simulink model "fo_FTSM"  (R2022b)
settings: Solver=VariableStepAuto  StartTime=0.0  StopTime=10.0  RelTol=1e-3
libraries: fod x2
settings Model: Creator=张倬境  LastModifiedBy=张倬境
settings DebuggingCC: MaskedZcDiagnostic=none  IgnoredZcDiagnostic=none

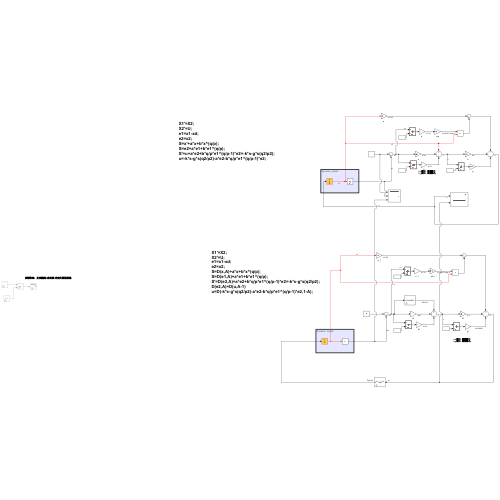
[thumbnail: Simulink's stored preview of the top-level diagram]
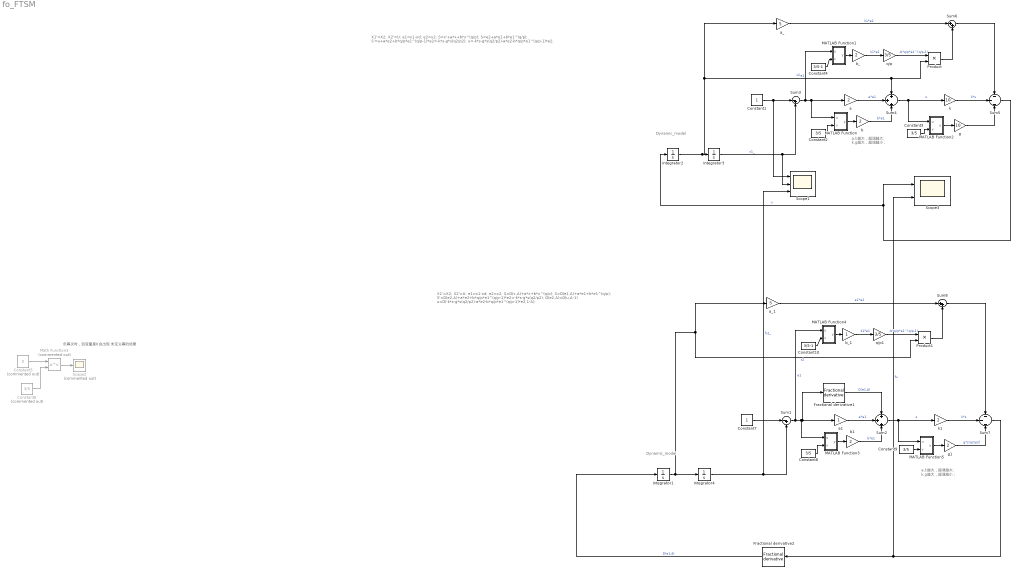
== system fo_FTSM ==
  note: a,b越大，超调越大;
      | k,g越大，超调越小；
  note: 负幂次时，自变量是0会出现 未定义幂的结果
  note: X1'=X2;
      | X2'=U;
      | e1=x1-xd;
      | e2=x2;
      | S=x'+a*x+b*x^(q/p);
      | S=e2+a*e1+b*e1^(q/p);
      | S'=u+a*e2+b*q/p*e1^(q/p-1)*e2=-k*s-g*s(q2/p2);
      | u=-k*s-g*s(q2/p2)-a*e2-b*q/p*e1^(q/p-1)*e2;
  note: Dynamic_model
  note: Dynamic_model
  note: a,b越大，超调越大;
      | k,g越大，超调越小；
  note: X1'=X2;
      | X2'=U;
      | e1=x1-xd;
      | e2=x2;
      | S=D(x,A)+a*x+b*x^(q/p);
      | S=D(e1,A)+a*e1+b*e1^(q/p);
      | S'=D(e2,A)+a*e2+b*q/p*e1^(q/p-1)*e2=-k*s-g*s(q2/p2);
      | D(e2,A)=D(u,A-1)
      | u=D(-k*s-g*s(q2/p2)-a*e2-b*q/p*e1^(q/p-1)*e2,1-A);
  Constant1 : Constant
  Constant10 : Constant  Value=3/5-1
  Constant{2..3,8..9} (4 alike) : Constant  Value=3/5
  Constant4 : Constant  Value=3/5-1
  Constant5 : Constant  Commented=on  Value=0
  Constant6 : Constant  Commented=on  Value=3/5
  Constant7 : Constant
  Fractional derivative1 : fod/Fractional derivative  gam=0.5  ww=[0.001; 1000]  n=5  nFod=off
      settings: SourceProductName=FOMCON Toolbox
  Fractional derivative2 : fod/Fractional derivative  gam=0.5  ww=[0.001; 1000]  n=5  nFod=off
      settings: SourceProductName=FOMCON Toolbox
  Integrator{1..4} (4 alike) : Integrator
  MATLAB Function : MATLAB Function  TreatAsAtomicUnit=on
  MATLAB Function1 : MATLAB Function  TreatAsAtomicUnit=on
  MATLAB Function2 : MATLAB Function  TreatAsAtomicUnit=on
  MATLAB Function3 : MATLAB Function  TreatAsAtomicUnit=on
  MATLAB Function4 : MATLAB Function  TreatAsAtomicUnit=on
  MATLAB Function5 : MATLAB Function  TreatAsAtomicUnit=on
  Math Function3 : Math  Commented=on  Operator=pow
  Product : Product
  Product1 : Product
  Scope1 : Scope  NumInputPorts=3
  Scope2 : Scope  Commented=on
  Scope3 : Scope  NumInputPorts=2
  Sum1 : Sum  Inputs=|-+
  Sum2 : Sum  Inputs=+|+|+
  Sum3 : Sum  Inputs=|-+
  Sum4 : Sum  Inputs=+|+|+
  Sum5 : Sum  Inputs=-|-|-
  Sum6 : Sum  Inputs=|++
  Sum7 : Sum  Inputs=-|-|-
  Sum8 : Sum  Inputs=|++
  a : Gain  Gain=2
  a1 : Gain
  a_ : Gain  Gain=5
  a_1 : Gain  Gain=5
  b : Gain  Gain=2
  b1 : Gain  Gain=2
  b_ : Gain  Gain=2
  b_1 : Gain
  g : Gain  Gain=10
  g1 : Gain  Gain=2
  k : Gain  Gain=10
  k1 : Gain  Gain=2
  q/p : Gain  Gain=3/5
  q/p1 : Gain  Gain=3/5
  wires:
  Sum5/1 -> Scope3/1, Integrator2/1  "u"
  Integrator2/1 -> a_/1, Product/2, Sum4/1, Integrator3/1  "x2"
  Integrator3/1 -> Scope1/2, Sum3/2  "x1_"
  a/1 -> Sum4/2  "a*e1"
  g/1 -> Sum5/3
  Constant1/1 -> Scope1/1, Sum3/1
  Constant2/1 -> MATLAB Function/2(v)
  MATLAB Function/1(y) -> b/1
  b/1 -> Sum4/3  "b*e1"
  k/1 -> Sum5/2  "k*s"
  Sum4/1 -> MATLAB Function2/1(u), k/1  "s"
  Constant3/1 -> MATLAB Function2/2(v)
  MATLAB Function2/1(y) -> g/1
  a_/1 -> Sum6/1  "k1*e2"
  Sum6/1 -> Sum5/1
  MATLAB Function1/1(y) -> b_/1
  Sum3/1 -> MATLAB Function1/1(u), MATLAB Function/1(u), a/1  "e1"
  b_/1 -> q/p/1  "k1*e1"
  Constant4/1 -> MATLAB Function1/2(v)
  q/p/1 -> Product/1  "-b*q/p*e1^(q/p-1)"
  Product/1 -> Sum6/2
  Constant5/1 -> Math Function3/1
  Constant6/1 -> Math Function3/2
  Math Function3/1 -> Scope2/1
  MATLAB Function5/1(y) -> g1/1
  Constant8/1 -> MATLAB Function3/2(v)
  a_1/1 -> Sum8/1  "a1*e2"
  b_1/1 -> q/p1/1  "k1*e1"
  Product1/1 -> Sum8/2
  q/p1/1 -> Product1/1  "-b*q/p*e1^(q/p-1)"
  Constant10/1 -> MATLAB Function4/2(v)
  Constant7/1 -> Sum1/1
  MATLAB Function3/1(y) -> b1/1
  MATLAB Function4/1(y) -> b_1/1
  g1/1 -> Sum7/3  "g*s(q2/p2)"
  Sum8/1 -> Sum7/1
  Integrator1/1 -> Product1/2, a_1/1, Integrator4/1  "x2"
  Sum1/1 -> MATLAB Function4/1(u), MATLAB Function3/1(u), Fractional derivative1/1, a1/1  "e1"
  Integrator4/1 -> Scope1/3, Sum1/2  "fx1_"
  a1/1 -> Sum2/2  "a*e1"
  Sum2/1 -> MATLAB Function5/1(u), k1/1  "s"
  k1/1 -> Sum7/2  "k*s"
  Constant9/1 -> MATLAB Function5/2(v)
  Sum7/1 -> Scope3/2, Fractional derivative2/1  "fu"
  b1/1 -> Sum2/3  "b*e1"
  Fractional derivative1/1 -> Sum2/1  "D(e1,A)"
  Fractional derivative2/1 -> Integrator1/1  "D(e1,A)"

== matlab function fo_FTSM/MATLAB Function ==
  data: u input; y output; v input
function y = fcn(u,v)
if u==0
    y=0;
else
    y=abs(u)^(v)*sign(u);
end
end

== matlab function fo_FTSM/MATLAB Function1 ==
  data: u input; y output; v input
function y = fcn(u,v)
if u==0
    y=0;
else
    y=abs(u)^(v)*sign(u);
end
end

== matlab function fo_FTSM/MATLAB Function2 ==
  data: u input; y output; v input
function y = fcn(u,v)
if u==0
    y=0;
else
    y=abs(u)^(v)*sign(u);
end
end

== matlab function fo_FTSM/MATLAB Function4 ==
  data: u input; y output; v input
function y = fcn(u,v)
if u==0
    y=0;
else
    y=abs(u)^(v)*sign(u);
end
end

== matlab function fo_FTSM/MATLAB Function5 ==
  data: u input; y output; v input
function y = fcn(u,v)
if u==0
    y=0;
else
    y=abs(u)^(v)*sign(u);
end
end

== matlab function fo_FTSM/MATLAB Function3 ==
  data: u input; y output; v input
function y = fcn(u,v)
if u==0
    y=0;
else
    y=abs(u)^(v)*sign(u);
end
end
